simulink model "AdaptiveMPC"  (R2022b)
settings: Solver=VariableStepAuto  StartTime=0.0  StopTime=40  FixedStep=0.02  RelTol=1e-5
values from neighbouring files (symbols this model uses):
  Matlab_version = str2double(r_temp___(1))    [3T_articulation_soft_terrain.m]
  Plant_inputs_num = r_temp___(1)    [3T_articulation_soft_terrain.m]
  Plant_outputs_num = r_temp___(1)    [3T_articulation_soft_terrain.m]
  RecurDyn_controltimestep = 1.e-003    (= 0.001)    [3T_articulation_soft_terrain.m]
  RecurDyn_CoSim = 'D:\Program Files\FunctionBay, Inc\RecurDyn V9R1\Toolkits\Controls\Simulink30\'    [3T_articulation_soft_terrain.m]
  RecurDyn_model = '3T_articulation_soft_terrain'    [3T_articulation_soft_terrain.m]
  RecurDyn_model_n = r_temp___(2)    [3T_articulation_soft_terrain.m]
undefined symbols (not defined in the file or in its folder): magnitude, val
libraries: mpclib x2
settings Model: PacingRate=3  Creator=HU  LastModifiedBy=HU
settings DebuggingCC: UnconnectedInputMsg=warning  UnconnectedOutputMsg=warning  UnconnectedLineMsg=warning  SFMachineParentedDataDiag=warning
settings ModelReferenceCC: EnableRefExpFcnMdlSchedulingChecks=on
settings RTWCC: DLArmComputeVersion=19.05

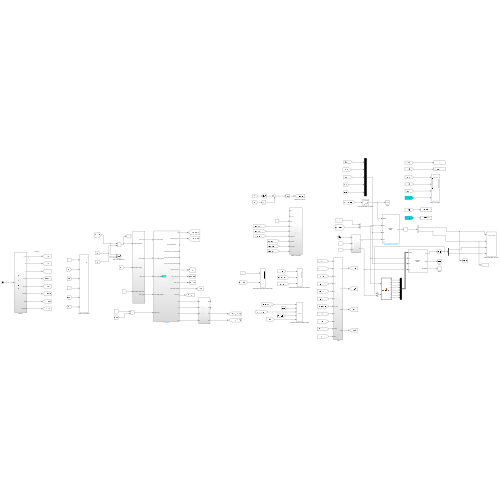
[thumbnail: Simulink's stored preview of the top-level diagram]
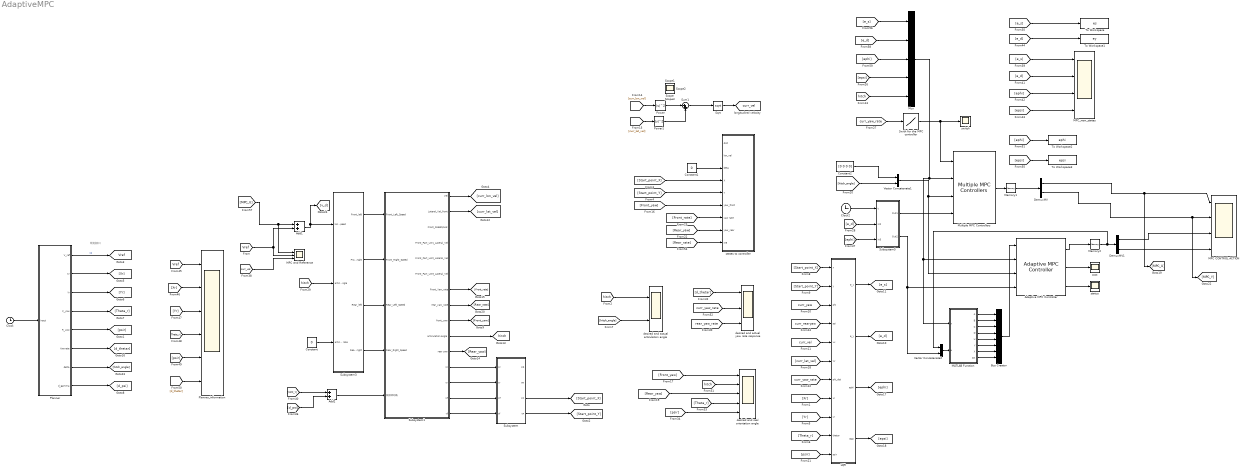
== system AdaptiveMPC ==
  note: 规划接口
  Adaptive MPC Controller : mpclib/Adaptive MPC Controller  SCDEnableBlockLinearizationSpecification=on  mpcobj=mpcobj_M_27  enable_value=0  updateMPCinCallerWorkspace=on  md_inport=on  mv_inport=off  uref_inport=off  return_cost=on  return_mvseq=off  return_qpstatus=on  return_xseq=off  return_state=off  return_ovseq=off  state_inport=off  isltv_plant=off  umin_inport=off  umax_inport=off  ymin_inport=off  ymax_inport=off  cc_inport=off  ywt_inport=off  uwt_inport=off  duwt_inport=off  rhoeps_inport=off  pm_inport=off  MaximumP=10  HorizonChoice=FixedHorizon  BlockDataType=double  SampleTimeInherited=off  switch_inport=off
  Add1 : Sum
  Add2 : Sum
  Bus Creator : BusCreator  Inputs=8
  Clock : Clock
  Clock2 : Clock
  Constant : Constant  Value=0
  Constant1 : Constant  Value=0
  Constant2 : Constant  Value=[0 0 0 0]
  DemuxMV : Demux  Outputs=2
  DemuxMV1 : Demux  Outputs=2
  LQR : Subsystem
  MATLAB Function : MATLAB Function  TreatAsAtomicUnit=on
  MPC CONTROL ACTION : Scope  NumInputPorts=4
  MPC and Reference : Scope  NumInputPorts=3
  MPC_new_states : Scope  NumInputPorts=4
  Memory1 : Memory
  Memory2 : Memory
  Multiple MPC Controllers : mpclib/Multiple MPC Controllers  mpcobjs={'mpcobj_L_21','mpcobj_M_21','mpcobj_H_21'}  x0s={'[]','[]','[]'}  Nmpc=1  theMPC=1  nmv=1  nmo=1  nmd=1  nts=1  md_inport_multiple=on  mv_inport_multiple=off  uref_inport_multiple=off  return_cost_multiple=off  return_mvseq_multiple=off  return_qpstatus_multiple=off  return_xseq_multiple=off  return_state_multiple=off  return_ovseq_multiple=off  state_inport_multiple=off  umin_inport_multiple=off  umax_inport_multiple=off  ymin_inport_multiple=off  ymax_inport_multiple=off  ywt_inport_multiple=off  uwt_inport_multiple=off  duwt_inport_multiple=off  rhoeps_inport_multiple=off  BlockDataType_multiple=double  SampleTimeInherited_multiple=off
  Mux : Mux  Inputs=5
  Planner : Subsystem
  Planner_information : Scope  NumInputPorts=6
  Power : Math  Operator=magnitude^2
  Power1 : Math  Operator=magnitude^2
  Sqrt : Sqrt
  Subsystem : Subsystem
  Subsystem1 : Subsystem
  Subsystem3 : Subsystem
  Subsystem5 : Subsystem
  Sum1 : Sum  Inputs=|++
  Swith for the MPC controller : Lookup_n-D  NumberOfTableDimensions=1  BreakpointsForDimension1="[-0.5  0  0.5]"  BreakpointsForDimension1FirstPoint=-0.1  BreakpointsForDimension1Spacing=0.1  Table="[1  2  3]"  InterpMethod=Nearest  InternalRulePriority=Speed  RndMeth=Simplest
  To Workspace : ToWorkspace  VariableName=es  SaveFormat=Timeseries  SampleTime=-1
  To Workspace1 : ToWorkspace  VariableName=ey  SaveFormat=Timeseries  SampleTime=-1
  To Workspace2 : ToWorkspace  VariableName=ephi  SaveFormat=Timeseries  SampleTime=-1
  To Workspace3 : ToWorkspace  VariableName=epsi  SaveFormat=Timeseries  SampleTime=-1
  Vector Concatenate1 : Concatenate
  Vector Concatenate2 : Concatenate  Mode=Multidimensional array  ConcatenateDimension=2
  cost : Scope
  desired and actual articulation angle : Scope  NumInputPorts=2
  desired and actual yaw rate response : Scope  NumInputPorts=3
  desired and real orientation angle : Scope  NumInputPorts=5
  states to controller : Subsystem
  status : Scope
  switch : Scope
  Scope{,1..3} (4 alike) : Scope
  tag scope: Vref=global, curr_vel=global, hitch=global
  wires:
  [Start_point_Y] -> states to controller/5(Y)
  LQR/2(e_y) -> [e_d]
  LQR/1(e_x) -> [e_s]
  Planner/1(V_ref) -> [Vref]  "vp"
  [Xr] -> LQR/8(xr)
  [Theta_r] -> LQR/10(thetar)
  Planner/4(F_yaw) -> [Theta_r]
  [curr_lat_vel] -> LQR/6(vy)
  Planner/3(Yr) -> [Yr]
  Sum1/1 -> Sqrt/1
  [curr_yaw_rate] -> LQR/7(phi_dot)
  [curr_vel] -> LQR/5(vx)
  [curr_yaw] -> LQR/3(phi)
  [Start_point_Y] -> LQR/2(y)
  [Start_point_X] -> LQR/1(x)
  [Yr] -> LQR/9(yr)
  Planner/2(Xr) -> [Xr]
  Power1/1 -> Sum1/2
  Constant1/1 -> states to controller/3(beta)
  Power/1 -> Sum1/1
  [Start_point_X] -> states to controller/4(X)
  Planner/6(Yawrate) -> [d_thetar]
  Planner/5(R_yaw) -> [psir]
  [psir] -> LQR/11(psir)
  [curr_rearyaw] -> LQR/4(psi)
  LQR/3(ephi) -> [ephi]
  LQR/4(epsi) -> [epsi]
  [d_thetar] -> desired and actual yaw rate response/1
  [Theta_r] -> desired and real orientation angle/4
  [psir] -> desired and real orientation angle/5
  [curr_yaw_rate] -> desired and actual yaw rate response/2
  [rear_yaw_rate] -> desired and actual yaw rate response/3
  [Front_yaw] -> desired and real orientation angle/1
  [Rear_yaw] -> desired and real orientation angle/3
  [e_s] -> MPC_new_states/1
  [e_d] -> MPC_new_states/2
  [ephi] -> MPC_new_states/3
  [epsi] -> MPC_new_states/4
  Subsystem1/2(Lateral_Vel_front) -> [curr_lat_vel]
  Subsystem3/1(Front_left) -> Subsystem1/1("Front_Left_Speed ")
  Subsystem3/2(Front_right) -> Subsystem1/2(Front_Right_Speed)
  Subsystem3/3(Rear_left) -> Subsystem1/3("Rear_Left_Speed  ")
  Subsystem3/4(Rear_right) -> Subsystem1/4("Rear_Right_Speed ")
  Subsystem1/12(Xr) -> Subsystem/1(Xr)
  Subsystem1/13(Yr) -> Subsystem/2(Yr)
  Subsystem1/14(Xf) -> Subsystem/3(Xf)
  Subsystem1/15(Yf) -> Subsystem/4(Yf)
  Subsystem1/1(Vel) -> [curr_lon_vel]
  [curr_lat_vel] -> Power1/1
  [curr_lon_vel] -> Power/1
  Subsystem1/9(front_yaw) -> [Front_yaw]
  [Front_yaw] -> states to controller/6(yaw_front)
  Subsystem1/11(rear yaw) -> [Rear_yaw]
  [Rear_yaw] -> states to controller/8(yaw_rear)
  Subsystem1/7(Front_Yaw_rate) -> [Front_rate]
  [Front_rate] -> states to controller/7(yaw rate)
  Subsystem1/8(rear_yaw_rate) -> [Rear_rate]
  Subsystem1/10(articulation angle) -> [hitch]
  [hitch] -> desired and real orientation angle/2
  [Vref] -> Planner_information/1
  [Yr] -> Planner_information/3
  [Theta_r] -> Planner_information/4
  [psir] -> Planner_information/5
  [d_thetar] -> Planner_information/6
  Planner/7(delta) -> [hitch_angle]
  [Xr] -> Planner_information/2
  Sqrt/1 -> [curr_vel]
  [hitch] -> Subsystem3/2(articulation angle)
  [Rear_rate] -> states to controller/9(In9)
  [ephi] -> Mux/3
  [hitch] -> Mux/5
  [e_d] -> Mux/2
  [e_s] -> Mux/1
  [MPC_U] -> Add1/1, MPC and Reference/1
  [Vref] -> Add1/2, MPC and Reference/2
  [epsi] -> Mux/4
  Mux/1 -> Multiple MPC Controllers/2, MATLAB Function/1(x), Adaptive MPC Controller/2
  Multiple MPC Controllers/1 -> Memory1/1
  Memory1/1 -> DemuxMV/1
  Swith for the MPC controller/1 -> Multiple MPC Controllers/1, switch/1
  Subsystem/4(YF) -> [Start_point_Y]
  Subsystem/3(XF) -> [Start_point_X]
  [hitch] -> desired and actual articulation angle/1
  [hitch_angle] -> desired and actual articulation angle/2
  Subsystem5/1(Out1) -> Multiple MPC Controllers/4
  [hitch_angle] -> Vector Concatenate1/2
  Constant2/1 -> Vector Concatenate1/1
  Clock2/1 -> Subsystem5/1(t)
  Vector Concatenate1/1 -> Multiple MPC Controllers/3, Adaptive MPC Controller/3
  MATLAB Function/1(A) -> Bus Creator/1
  MATLAB Function/2(B) -> Bus Creator/2
  MATLAB Function/3(C) -> Bus Creator/3
  MATLAB Function/4(D) -> Bus Creator/4
  MATLAB Function/5(U) -> Bus Creator/5
  MATLAB Function/6(Y) -> Bus Creator/6
  MATLAB Function/7(X) -> Bus Creator/7
  MATLAB Function/8(DX) -> Bus Creator/8
  Bus Creator/1 -> Adaptive MPC Controller/1
  Adaptive MPC Controller/1 -> Memory2/1
  DemuxMV1/1 -> MPC CONTROL ACTION/3
  DemuxMV1/2 -> MPC CONTROL ACTION/4
  Vector Concatenate2/1 -> MATLAB Function/2(u)
  Planner/8(d_gamma) -> [d_psi]
  [curr_yaw_rate] -> Swith for the MPC controller/1
  Memory2/1 -> Vector Concatenate2/1, DemuxMV1/1
  [e_d] -> Subsystem5/2(In2)
  [ephi] -> Subsystem5/3(In3)
  Adaptive MPC Controller/2 -> cost/1
  Adaptive MPC Controller/3 -> status/1
  [curr_vel] -> MPC and Reference/3
  Constant/1 -> Subsystem3/3(articulation angle rate)
  Add1/1 -> Subsystem3/1(longitudinal speed), [v_d]
  Subsystem5/2(Out2) -> Adaptive MPC Controller/4, Vector Concatenate2/2
  Clock/1 -> Planner/1(Input)
  [e_s] -> To Workspace/1
  [e_d] -> To Workspace1/1
  [ephi] -> To Workspace2/1
  [epsi] -> To Workspace3/1
  [MPC_Y] -> Add2/1
  Add2/1 -> Subsystem1/5("铰接转动角            ")
  [d_psi] -> Add2/2
  DemuxMV/1 -> [MPC_U], MPC CONTROL ACTION/1
  DemuxMV/2 -> [MPC_Y], MPC CONTROL ACTION/2

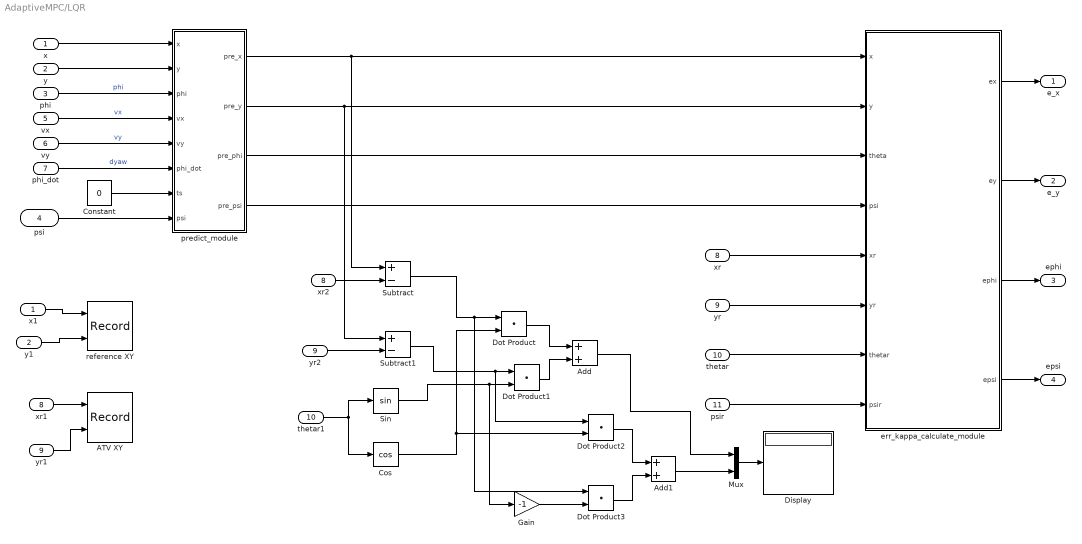
== system AdaptiveMPC/LQR ==
  x : Inport
  y : Inport  Port=2
  phi : Inport  Port=3
  psi : Inport  Port=4
  vx : Inport  Port=5
  vy : Inport  Port=6
  phi_dot : Inport  Port=7
  xr : Inport  Port=8
  yr : Inport  Port=9
  thetar : Inport  Port=10
  psir : Inport  Port=11
  ATV XY : Record  FileSettingsInternal="{\"entries\":[{\"content\":{\"excelSettings\":{\"content\":{},\"type\":\"Streamout.ExcelSettings\"}},\"type\":\"Streamout.FileSettingStorage\",\"uuid\":\"7d4ff071-c011-4d00-aaca-92aa85f924c6\"}],\"packageUris\":[\"http://schema.mathworks.com/mf0/streamout_blocks/R2020a\"],\"version\":\"1.0\"}"  Layout=[1 1]  SignalsInternal="{\"entries\":[{\"content\":{\"signals\":[{\"content\":{\"blockPath\":[\"AdaptiveMPC_only_MPC/LQR/ATV XY\"],\"channel\":[],\"dimensions\":[1],\"domain\":\"AdaptiveMPC_only_MPC/LQR/ATV XY\",\"lineColor\":\"#a2142f\",\"plots\":[1],\"port\":1,\"sid\":[\"\"],\"signalID\":165725,\"signalName\":\"xr1\"},\"type\":\"RecordBlkView.Signal\",\"uuid\":\"68c8aef4-2586-4868-bddc-4b1de75c0796\"},{\"content\":{\"blockPath\":[\"AdaptiveMPC_only_MPC/LQR/ATV XY\"],\"channel\":[],\"dimensions\":[1],\"domain\":\"AdaptiveMPC_only_MPC/LQR/ATV XY\",\"lineColor\":\"#139fff\",\"plots\":[1],\"port\":2,\"sid\":[\"\"],\"signalID\":165729,\"signalName\":\"yr1\"},\"type\":\"RecordBlkView.Signal\",\"uuid\":\"206c790a-a246-4103-b7c9-0af210733676\"}]},\"type\":\"RecordBlkView.InputSignals\",\"uuid\":\"6523171a-3a0a-4dbe-b18c-2b5d012fbce6\"}],\"packageUris\":[\"http://schema.mathworks.com/mf0/streamout_blocks/R2020a\"],\"version\":\"1.0\"}"  VisualizationBindings="{\"xyplotplugin\":{\"info\":[{\"series\":[{\"bindingParametersList\":[{\"parameter\":\"X-Axis\",\"signalID\":165725,\"signalName\":\"xr1\"},{\"parameter\":\"Y-Axis\",\"signalID\":165729,\"signalName\":\"yr1\"}],\"seriesID\":583}],\"subplotID\":1}]}}"  CompatibilityTag=XY  st=-1
  Add : Sum
  Add1 : Sum
  Constant : Constant  Value=0
  Cos : Trigonometry  Operator=cos
  Display : Display
  Dot Product{,1..3} (4 alike) : DotProduct  OutDataTypeStr=Inherit: Inherit via internal rule
  Gain : Gain  Gain=-1
  Mux : Mux  Inputs=2
  Sin : Trigonometry
  Subtract : Sum  Inputs=+-
  Subtract1 : Sum  Inputs=+-
  err_kappa_calculate_module : MATLAB Function  TreatAsAtomicUnit=on
  predict_module : MATLAB Function  TreatAsAtomicUnit=on
  reference XY : Record  FileSettingsInternal="{\"entries\":[{\"content\":{\"excelSettings\":{\"content\":{},\"type\":\"Streamout.ExcelSettings\"}},\"type\":\"Streamout.FileSettingStorage\",\"uuid\":\"01dd9b82-04e5-459d-9b91-d9a9579cc2c9\"}],\"packageUris\":[\"http://schema.mathworks.com/mf0/streamout_blocks/R2020a\"],\"version\":\"1.0\"}"  Layout=[1 1]  SignalsInternal="{\"entries\":[{\"content\":{\"signals\":[{\"content\":{\"blockPath\":[\"AdaptiveMPC_only_MPC/LQR/reference XY\"],\"channel\":[],\"dimensions\":[1],\"domain\":\"AdaptiveMPC_only_MPC/LQR/reference XY\",\"lineColor\":\"#a2142f\",\"plots\":[1],\"port\":1,\"sid\":[\"\"],\"signalID\":165733,\"signalName\":\"x1\"},\"type\":\"RecordBlkView.Signal\",\"uuid\":\"15320c6c-986b-4afd-bf62-20c31eac0383\"},{\"content\":{\"blockPath\":[\"AdaptiveMPC_only_MPC/LQR/reference XY\"],\"channel\":[],\"dimensions\":[1],\"domain\":\"AdaptiveMPC_only_MPC/LQR/reference XY\",\"lineColor\":\"#139fff\",\"plots\":[1],\"port\":2,\"sid\":[\"\"],\"signalID\":165737,\"signalName\":\"y1\"},\"type\":\"RecordBlkView.Signal\",\"uuid\":\"756ffe9f-769c-4c77-bafa-21ea174eeee0\"}]},\"type\":\"RecordBlkView.InputSignals\",\"uuid\":\"98c54ad5-dfe3-4874-ac3d-5744926d3a13\"}],\"packageUris\":[\"http://schema.mathworks.com/mf0/streamout_blocks/R2020a\"],\"version\":\"1.0\"}"  VisualizationBindings="{\"xyplotplugin\":{\"info\":[{\"series\":[{\"bindingParametersList\":[{\"parameter\":\"X-Axis\",\"signalID\":165733,\"signalName\":\"x1\"},{\"parameter\":\"Y-Axis\",\"signalID\":165737,\"signalName\":\"y1\"}],\"seriesID\":16425}],\"subplotID\":1}]}}"  CompatibilityTag=XY  st=-1
  thetar1 : InportShadow  Port=10
  x1 : InportShadow
  xr1 : InportShadow  Port=8
  xr2 : InportShadow  Port=8
  y1 : InportShadow  Port=2
  yr1 : InportShadow  Port=9
  yr2 : InportShadow  Port=9
  e_x : Outport  VectorParamsAs1DForOutWhenUnconnected=off
  e_y : Outport  Port=2  VectorParamsAs1DForOutWhenUnconnected=off
  ephi : Outport  Port=3  VectorParamsAs1DForOutWhenUnconnected=off
  epsi : Outport  Port=4  VectorParamsAs1DForOutWhenUnconnected=off
  wires:
  vy/1 -> predict_module/5(vy)  "vy"
  x/1 -> predict_module/1(x)
  predict_module/2(pre_y) -> Subtract1/1, err_kappa_calculate_module/2(y)
  phi_dot/1 -> predict_module/6(phi_dot)  "dyaw"
  vx/1 -> predict_module/4(vx)  "vx"
  y/1 -> predict_module/2(y)
  phi/1 -> predict_module/3(phi)  "phi"
  Constant/1 -> predict_module/7(ts)
  predict_module/1(pre_x) -> Subtract/1, err_kappa_calculate_module/1(x)
  predict_module/3(pre_phi) -> err_kappa_calculate_module/3(theta)
  xr/1 -> err_kappa_calculate_module/5(xr)
  yr/1 -> err_kappa_calculate_module/6(yr)
  thetar/1 -> err_kappa_calculate_module/7(thetar)
  psi/1 -> predict_module/8(psi)
  predict_module/4(pre_psi) -> err_kappa_calculate_module/4(psi)
  psir/1 -> err_kappa_calculate_module/8(psir)
  err_kappa_calculate_module/2(ey) -> e_y/1
  err_kappa_calculate_module/1(ex) -> e_x/1
  xr1/1 -> ATV XY/1
  yr1/1 -> ATV XY/2
  x1/1 -> reference XY/1
  y1/1 -> reference XY/2
  err_kappa_calculate_module/4(epsi) -> epsi/1
  err_kappa_calculate_module/3(ephi) -> ephi/1
  xr2/1 -> Subtract/2
  yr2/1 -> Subtract1/2
  thetar1/1 -> Cos/1, Sin/1
  Subtract/1 -> Dot Product/1, Dot Product3/1
  Cos/1 -> Dot Product2/2, Dot Product/2
  Subtract1/1 -> Dot Product2/1, Dot Product1/1
  Sin/1 -> Gain/1, Dot Product1/2
  Dot Product/1 -> Add/1
  Dot Product1/1 -> Add/2
  Gain/1 -> Dot Product3/2
  Dot Product2/1 -> Add1/1
  Dot Product3/1 -> Add1/2
  Add/1 -> Mux/1
  Add1/1 -> Mux/2
  Mux/1 -> Display/1

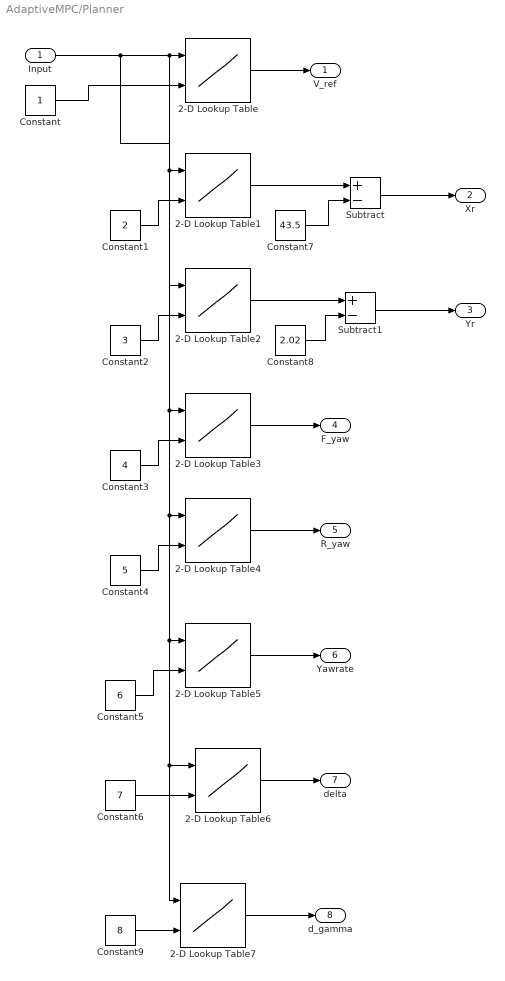
== system AdaptiveMPC/Planner ==
  Input : Inport
  2-D Lookup Table{,1..7} (8 alike) : Lookup_n-D  BreakpointsForDimension1=t  BreakpointsForDimension2=[1:8]  Table=val  InternalRulePriority=Speed  RndMeth=Simplest
      settings: InputPortMap=u0,u1
  Constant : Constant
  Constant1 : Constant  Value=2
  Constant2 : Constant  Value=3
  Constant3 : Constant  Value=4
  Constant4 : Constant  Value=5
  Constant5 : Constant  Value=6
  Constant6 : Constant  Value=7
  Constant7 : Constant  Value=43.5
  Constant8 : Constant  Value=2.02
  Constant9 : Constant  Value=8
  Subtract : Sum  Inputs=+-
  Subtract1 : Sum  Inputs=+-
  V_ref : Outport
  Xr : Outport  Port=2
  Yr : Outport  Port=3
  F_yaw : Outport  Port=4
  R_yaw : Outport  Port=5
  Yawrate : Outport  Port=6
  delta : Outport  Port=7
  d_gamma : Outport  Port=8
  wires:
  2-D Lookup Table6/1 -> delta/1
  Constant6/1 -> 2-D Lookup Table6/2
  Constant5/1 -> 2-D Lookup Table5/2
  2-D Lookup Table5/1 -> Yawrate/1
  Constant3/1 -> 2-D Lookup Table3/2
  Constant4/1 -> 2-D Lookup Table4/2
  2-D Lookup Table3/1 -> F_yaw/1
  Constant1/1 -> 2-D Lookup Table1/2
  2-D Lookup Table/1 -> V_ref/1
  Constant/1 -> 2-D Lookup Table/2
  Constant2/1 -> 2-D Lookup Table2/2
  Input/1 -> 2-D Lookup Table7/1, 2-D Lookup Table6/1, 2-D Lookup Table5/1, 2-D Lookup Table4/1, 2-D Lookup Table3/1, 2-D Lookup Table1/1, 2-D Lookup Table2/1, 2-D Lookup Table/1
  2-D Lookup Table4/1 -> R_yaw/1
  2-D Lookup Table1/1 -> Subtract/1
  Constant7/1 -> Subtract/2
  Subtract/1 -> Xr/1
  Subtract1/1 -> Yr/1
  Constant8/1 -> Subtract1/2
  2-D Lookup Table2/1 -> Subtract1/1
  Constant9/1 -> 2-D Lookup Table7/2
  2-D Lookup Table7/1 -> d_gamma/1

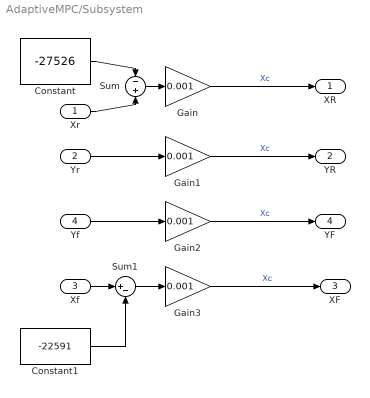
== system AdaptiveMPC/Subsystem ==
  Xr : Inport
  Yr : Inport  Port=2
  Xf : Inport  Port=3
  Yf : Inport  Port=4
  Constant : Constant  Value=-27526
  Constant1 : Constant  Value=-22591
  Gain{,1..3} (4 alike) : Gain  Gain=0.001
  Sum : Sum  Inputs=-+
  Sum1 : Sum  Inputs=|+-
  XR : Outport
  YR : Outport  Port=2
  XF : Outport  Port=3
  YF : Outport  Port=4
  wires:
  Gain/1 -> XR/1  "Xc"
  Xr/1 -> Sum/2
  Constant/1 -> Sum/1
  Sum/1 -> Gain/1
  Yr/1 -> Gain1/1
  Yf/1 -> Gain2/1
  Xf/1 -> Sum1/1
  Constant1/1 -> Sum1/2
  Sum1/1 -> Gain3/1
  Gain1/1 -> YR/1  "Xc"
  Gain3/1 -> XF/1  "Xc"
  Gain2/1 -> YF/1  "Xc"

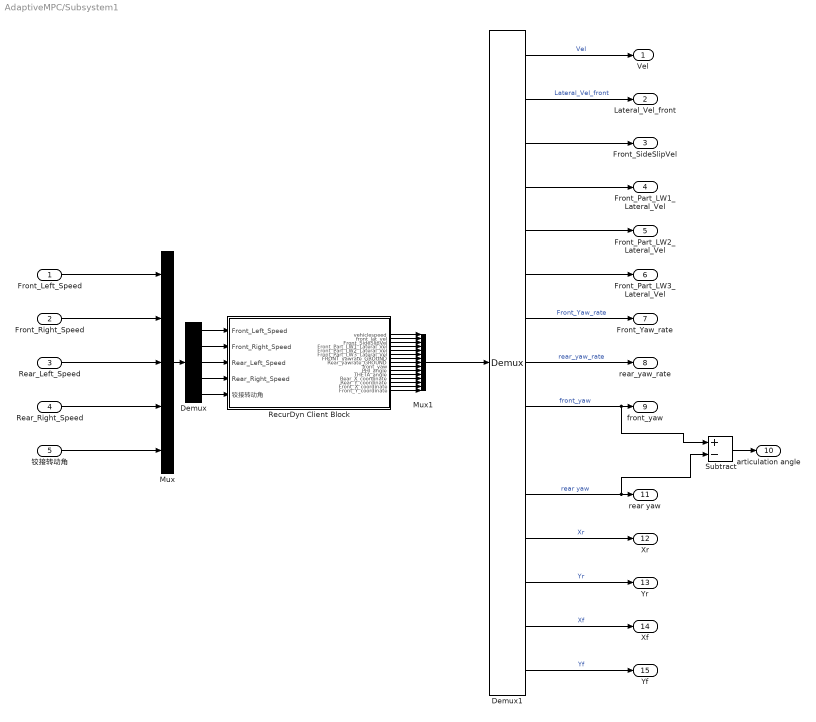
== system AdaptiveMPC/Subsystem1 ==
  "Front_Left_Speed " : Inport
  Front_Right_Speed : Inport  Port=2
  "Rear_Left_Speed  " : Inport  Port=3
  "Rear_Right_Speed " : Inport  Port=4
  "铰接转动角            " : Inport  Port=5
  Demux : Demux  Outputs=5
  Demux1 : Demux  Outputs=15
  Mux : Mux  Inputs=5
  Mux1 : Mux  Inputs=15
  RecurDyn Client Block : Subsystem
      mask Display: image(imread('RecurDyn_IF3x_Client.jpg'))
  Subtract : Sum  Inputs=+-
  Vel : Outport
  Lateral_Vel_front : Outport  Port=2
  "Front_SideSlipVel         " : Outport  Port=3
  Front_Part_LW1_Lateral_Vel : Outport  Port=4
  Front_Part_LW2_Lateral_Vel : Outport  Port=5
  Front_Part_LW3_Lateral_Vel : Outport  Port=6
  Front_Yaw_rate : Outport  Port=7
  rear_yaw_rate : Outport  Port=8
  front_yaw : Outport  Port=9
  articulation angle : Outport  Port=10
  rear yaw : Outport  Port=11
  Xr : Outport  Port=12
  Yr : Outport  Port=13
  Xf : Outport  Port=14
  Yf : Outport  Port=15
  wires:
  "Rear_Left_Speed  "/1 -> Mux/3
  Demux1/8 -> rear_yaw_rate/1  "rear_yaw_rate"
  Demux1/1 -> Vel/1  "Vel"
  Demux1/3 -> "Front_SideSlipVel         "/1
  Demux1/7 -> Front_Yaw_rate/1  "Front_Yaw_rate"
  Demux1/14 -> Xf/1  "Xf"
  Demux1/2 -> Lateral_Vel_front/1  "Lateral_Vel_front"
  Front_Right_Speed/1 -> Mux/2
  Demux1/13 -> Yr/1  "Yr"
  Demux1/12 -> Xr/1  "Xr"
  Demux1/15 -> Yf/1  "Yf"
  Demux1/4 -> Front_Part_LW1_Lateral_Vel/1
  "Front_Left_Speed "/1 -> Mux/1
  "Rear_Right_Speed "/1 -> Mux/4
  "铰接转动角            "/1 -> Mux/5
  Demux1/6 -> Front_Part_LW3_Lateral_Vel/1
  Demux1/5 -> Front_Part_LW2_Lateral_Vel/1
  Demux/1 -> RecurDyn Client Block/1("Front_Left_Speed ")
  Demux/2 -> RecurDyn Client Block/2(Front_Right_Speed)
  Demux/3 -> RecurDyn Client Block/3("Rear_Left_Speed  ")
  Demux/4 -> RecurDyn Client Block/4("Rear_Right_Speed ")
  Demux/5 -> RecurDyn Client Block/5("铰接转动角            ")
  Mux/1 -> Demux/1
  RecurDyn Client Block/1("vehiclespeed              ") -> Mux1/1
  RecurDyn Client Block/2("front_lat_vel             ") -> Mux1/2
  RecurDyn Client Block/3("Front_SideSlipVel         ") -> Mux1/3
  RecurDyn Client Block/4(Front_Part_LW1_Lateral_Vel) -> Mux1/4
  RecurDyn Client Block/5(Front_Part_LW2_Lateral_Vel) -> Mux1/5
  RecurDyn Client Block/6(Front_Part_LW3_Lateral_Vel) -> Mux1/6
  RecurDyn Client Block/7("FRONT_yawrate_GROUND      ") -> Mux1/7
  RecurDyn Client Block/8("Rear_yawrate_GROUND       ") -> Mux1/8
  RecurDyn Client Block/9("front_yaw                 ") -> Mux1/9
  RecurDyn Client Block/10("PHI_angle                 ") -> Mux1/10
  RecurDyn Client Block/11("THETA_angle               ") -> Mux1/11
  RecurDyn Client Block/12("Rear_X_coordinate         ") -> Mux1/12
  RecurDyn Client Block/13("Rear_Y_coordinate         ") -> Mux1/13
  RecurDyn Client Block/14("Front_X_coordinate        ") -> Mux1/14
  RecurDyn Client Block/15("Front_Y_coordinate        ") -> Mux1/15
  Mux1/1 -> Demux1/1
  Demux1/9 -> Subtract/1, front_yaw/1  "front_yaw"
  Demux1/11 -> Subtract/2, rear yaw/1  "rear yaw"
  Subtract/1 -> articulation angle/1

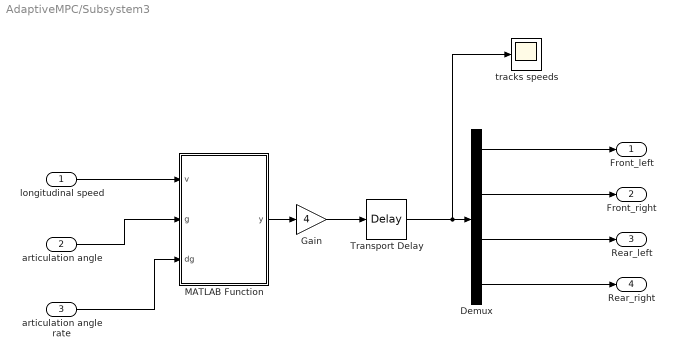
== system AdaptiveMPC/Subsystem3 ==
  longitudinal speed : Inport
  articulation angle : Inport  Port=2
  articulation angle rate : Inport  Port=3
  Demux : Demux
  Gain : Gain  Gain=4
  MATLAB Function : MATLAB Function  TreatAsAtomicUnit=on
  Transport Delay : TransportDelay  DelayTime=0.1
  tracks speeds : Scope
  Front_left : Outport
  Front_right : Outport  Port=2
  Rear_left : Outport  Port=3
  Rear_right : Outport  Port=4
  wires:
  articulation angle/1 -> MATLAB Function/2(g)
  MATLAB Function/1(y) -> Gain/1
  Gain/1 -> Transport Delay/1
  Demux/1 -> Front_left/1
  Demux/2 -> Front_right/1
  Demux/3 -> Rear_left/1
  Demux/4 -> Rear_right/1
  articulation angle rate/1 -> MATLAB Function/3(dg)
  Transport Delay/1 -> tracks speeds/1, Demux/1
  longitudinal speed/1 -> MATLAB Function/1(v)

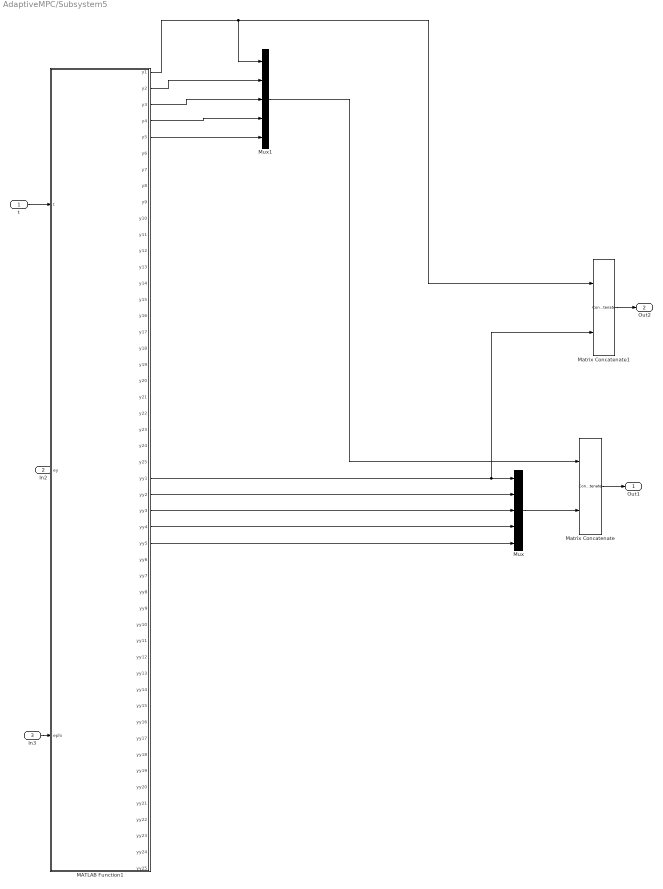
== system AdaptiveMPC/Subsystem5 ==
  t : Inport
  In2 : Inport  Port=2
  In3 : Inport  Port=3
  MATLAB Function1 : MATLAB Function  TreatAsAtomicUnit=on  SystemSampleTime=0.02
  Matrix Concatenate : Concatenate  Mode=Multidimensional array  ConcatenateDimension=2
  Matrix Concatenate1 : Concatenate  Mode=Multidimensional array  ConcatenateDimension=2
  Mux : Mux  Inputs=5
  Mux1 : Mux  Inputs=5
  Out1 : Outport
  Out2 : Outport  Port=2
  wires:
  MATLAB Function1/5(y5) -> Mux1/5
  Matrix Concatenate/1 -> Out1/1
  Mux/1 -> Matrix Concatenate/2
  MATLAB Function1/26(yy1) -> Matrix Concatenate1/2, Mux/1
  MATLAB Function1/29(yy4) -> Mux/4
  MATLAB Function1/3(y3) -> Mux1/3
  MATLAB Function1/4(y4) -> Mux1/4
  MATLAB Function1/1(y1) -> Matrix Concatenate1/1, Mux1/1
  MATLAB Function1/2(y2) -> Mux1/2
  MATLAB Function1/27(yy2) -> Mux/2
  MATLAB Function1/30(yy5) -> Mux/5
  MATLAB Function1/28(yy3) -> Mux/3
  Mux1/1 -> Matrix Concatenate/1
  t/1 -> MATLAB Function1/1(t)
  Matrix Concatenate1/1 -> Out2/1
  In2/1 -> MATLAB Function1/2(ey)
  In3/1 -> MATLAB Function1/3(ephi)

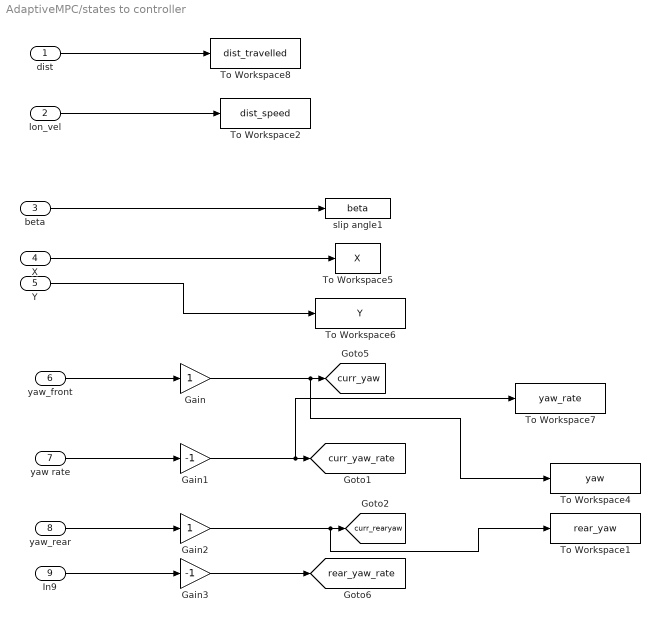
== system AdaptiveMPC/states to controller ==
  dist : Inport
  lon_vel : Inport  Port=2
  beta : Inport  Port=3
  X : Inport  Port=4
  Y : Inport  Port=5
  yaw_front : Inport  Port=6
  yaw rate : Inport  Port=7
  yaw_rear : Inport  Port=8
  In9 : Inport  Port=9
  Gain : Gain
  Gain1 : Gain  Gain=-1
  Gain2 : Gain
  Gain3 : Gain  Gain=-1
  To Workspace1 : ToWorkspace  VariableName=rear_yaw  SaveFormat=Timeseries  SampleTime=-1
  To Workspace2 : ToWorkspace  VariableName=dist_speed  SaveFormat=Timeseries  SampleTime=-1
  To Workspace4 : ToWorkspace  VariableName=yaw  SaveFormat=Timeseries  SampleTime=-1
  To Workspace5 : ToWorkspace  VariableName=X  SampleTime=-1
  To Workspace6 : ToWorkspace  VariableName=Y  SampleTime=-1
  To Workspace7 : ToWorkspace  VariableName=yaw_rate  SaveFormat=Timeseries  SampleTime=-1
  To Workspace8 : ToWorkspace  VariableName=dist_travelled  SaveFormat=Timeseries  SampleTime=-1
  slip angle1 : ToWorkspace  VariableName=beta  SaveFormat=Timeseries  SampleTime=-1
  tag scope: curr_rearyaw=global, curr_yaw=global, curr_yaw_rate=global, rear_yaw_rate=global
  wires:
  X/1 -> To Workspace5/1
  Y/1 -> To Workspace6/1
  beta/1 -> slip angle1/1
  yaw_front/1 -> Gain/1
  dist/1 -> To Workspace8/1
  lon_vel/1 -> To Workspace2/1
  yaw rate/1 -> Gain1/1
  Gain/1 -> To Workspace4/1, [curr_yaw]
  Gain1/1 -> To Workspace7/1, [curr_yaw_rate]
  Gain2/1 -> To Workspace1/1, [curr_rearyaw]
  yaw_rear/1 -> Gain2/1
  Gain3/1 -> [rear_yaw_rate]
  In9/1 -> Gain3/1

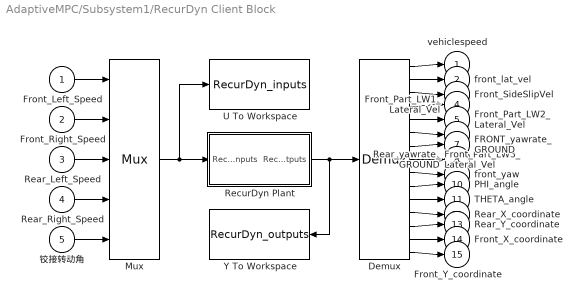
== system AdaptiveMPC/Subsystem1/RecurDyn Client Block ==
  "Front_Left_Speed " : Inport
  Front_Right_Speed : Inport  Port=2
  "Rear_Left_Speed  " : Inport  Port=3
  "Rear_Right_Speed " : Inport  Port=4
  "铰接转动角            " : Inport  Port=5
  Demux : Demux  Outputs=15
      settings: DisplayOption=none
  Mux : Mux  Inputs=5
  RecurDyn Plant : Subsystem  mask(Recurdyn/Plant){RecurDyn_model_name=RecurDyn_model, RecurDyn_controltimestep_=RecurDyn_controltimestep, RecurDyn_step_=10000, Waitingtime=1000, Matlab_version_=Matlab_version}
      mask prompts: RecurDyn_model_name "Model name"; RecurDyn_controltimestep_ "Sampling period"; RecurDyn_step_ "Step"; Waitingtime "Waiting time"; Matlab_version_ "Matlab version"
      mask help:
      | Simulate any Recurdyn Dynamics Model in Recurdyn/Solver
      | Plant inputs and Plant outputs are transfered every sampling time
      | Here, sampling time is determined by sampling period (Control time step)
      mask Display: disp( 'Dynamic Model' )
  U To Workspace : ToWorkspace  VariableName=RecurDyn_inputs
  Y To Workspace : ToWorkspace  VariableName=RecurDyn_outputs
  "vehiclespeed              " : Outport
  "front_lat_vel             " : Outport  Port=2
  "Front_SideSlipVel         " : Outport  Port=3
  Front_Part_LW1_Lateral_Vel : Outport  Port=4
  Front_Part_LW2_Lateral_Vel : Outport  Port=5
  Front_Part_LW3_Lateral_Vel : Outport  Port=6
  "FRONT_yawrate_GROUND      " : Outport  Port=7
  "Rear_yawrate_GROUND       " : Outport  Port=8
  "front_yaw                 " : Outport  Port=9
  "PHI_angle                 " : Outport  Port=10
  "THETA_angle               " : Outport  Port=11
  "Rear_X_coordinate         " : Outport  Port=12
  "Rear_Y_coordinate         " : Outport  Port=13
  "Front_X_coordinate        " : Outport  Port=14
  "Front_Y_coordinate        " : Outport  Port=15
  wires:
  "铰接转动角            "/1 -> Mux/5
  "Rear_Right_Speed "/1 -> Mux/4
  "Rear_Left_Speed  "/1 -> Mux/3
  Front_Right_Speed/1 -> Mux/2
  "Front_Left_Speed "/1 -> Mux/1
  Demux/15 -> "Front_Y_coordinate        "/1
  Demux/14 -> "Front_X_coordinate        "/1
  Demux/13 -> "Rear_Y_coordinate         "/1
  Demux/12 -> "Rear_X_coordinate         "/1
  Demux/11 -> "THETA_angle               "/1
  Demux/10 -> "PHI_angle                 "/1
  Demux/9 -> "front_yaw                 "/1
  Demux/8 -> "Rear_yawrate_GROUND       "/1
  Demux/7 -> "FRONT_yawrate_GROUND      "/1
  Demux/6 -> Front_Part_LW3_Lateral_Vel/1
  Demux/5 -> Front_Part_LW2_Lateral_Vel/1
  Demux/4 -> Front_Part_LW1_Lateral_Vel/1
  Demux/3 -> "Front_SideSlipVel         "/1
  Demux/2 -> "front_lat_vel             "/1
  Demux/1 -> "vehiclespeed              "/1
  Mux/1 -> U To Workspace/1, RecurDyn Plant/1(" RecurDyn_inputs")
  RecurDyn Plant/1(RecurDyn_outputs) -> Y To Workspace/1, Demux/1

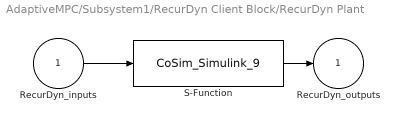
== system AdaptiveMPC/Subsystem1/RecurDyn Client Block/RecurDyn Plant ==
  " RecurDyn_inputs" : Inport
  S-Function : S-Function  FunctionName=CoSim_Simulink_9  Parameters=RecurDyn_controltimestep_,RecurDyn_model_name,RecurDyn_step_,Matlab_version_,RecurDyn_model_n,Plant_inputs_num,Plant_outputs_num,Waitingtime,RecurDyn_CoSim  SFunctionDeploymentMode=off  EnableBusSupport=off
  RecurDyn_outputs : Outport  InitialOutput=0
  wires:
  " RecurDyn_inputs"/1 -> S-Function/1
  S-Function/1 -> RecurDyn_outputs/1

== matlab function AdaptiveMPC/Subsystem3/MATLAB Function ==
  data: v input; y output; g input; dg input
function y = fcn(v, g, dg)
l=5;d=2.3;L1 = 2.6;L2 = 2.3; 
sg=sin(g); cg = L1+cos(g)*L2;c_g = 2*(L2+L1*cos(g));
t12 = v*sg/(2*cg);
t13 = v*dg*d*L1/(2*cg);
t21 = v*cos(g);
t22 = v*sg^2*L2/(c_g);
t23 = v*d*sg/c_g;
t24 = v*dg*L2*(2*L2*sg-d*cos(g))/c_g;
t25 = v*dg*L2*(2*L2*sg+d*cos(g))/c_g;
% y=[v+t12-t13;
%     v-t12+t13;
%     t21+t22+t23+t24;
%     t21+t22-t23+t25];
y  = [v;
      v;
      v*cos(g);
      v*cos(g)];

== matlab function AdaptiveMPC/MATLAB Function ==
  data: x input; u input; A output; B output; C output; D output; U output size=[4 1]; Y output size=[5 1]; X output size=[5 1]; DX output size=[5 1]
function [A,B,C,D,U,Y,X,DX] = adaptive_ATV(x,u)
[A,B,C,D,U,Y,X,DX] = ArticulatedVehicleModelDT32(x,u);

== matlab function AdaptiveMPC/LQR/err_kappa_calculate_module ==
  data: x input; y input; theta input; psi input; xr input; yr input; thetar input; ex output; ey output; ephi output; epsi output; psir input
function [ex,ey,ephi,epsi] = fcn(x,y,theta,psi,xr,yr,thetar,psir)
    
    tor=[cos(thetar);sin(thetar)];
    nor=[-sin(thetar);cos(thetar)];
    d_err=[x-xr;y-yr];
    ex=tor'*d_err;
    ey=nor'*d_err;

    %%%%%%%%%
    ephi = theta-thetar;
    epsi = psi-psir;
    %%%%%%%%%
    
    
    
    
    
    
    
    
    
    
    


end

== matlab function AdaptiveMPC/LQR/predict_module ==
  data: x input; pre_x output; y input; phi input; vx input; vy input; phi_dot input; ts input; pre_y output; pre_phi output; pre_psi output; psi input
function [pre_x,pre_y,pre_phi,pre_psi] = fcn(x,y,phi,vx,vy,phi_dot,ts, psi)
    pre_x=x+vx*ts*cos(phi)-vy*ts*sin(phi);
    pre_y=y+vy*ts*cos(phi)+vx*ts*sin(phi);
    pre_phi=phi+phi_dot*ts;
    pre_psi = psi + phi_dot*ts;
end

== matlab function AdaptiveMPC/Subsystem5/MATLAB Function1 ==
  data: t input double size=1; y1 output; y2 output; y3 output; y4 output; y5 output; y6 output; y7 output; y8 output; y9 output; y10 output; y11 output; y12 output; y13 output; y14 output; y15 output; y16 output; y17 output; y18 output; y19 output; y20 output; y21 output; y22 output; y23 output; y24 output; y25 output; yy1 output; yy2 output; yy3 output; yy4 output; yy5 output; yy6 output; yy7 output; yy8 output; yy9 output; yy10 output; yy11 output; yy12 output; yy13 output; yy14 output; yy15 output; yy16 output; yy17 output; yy18 output; yy19 output; yy20 output; yy21 output; yy22 output; yy23 output; yy24 output; yy25 output; ey input; ephi input
function [y1, y2, y3, y4, y5, y6, y7, y8, y9, y10, y11, y12, y13, y14, y15, y16, y17,y18, y19, y20, y21, y22, y23, y24, y25, yy1, yy2, yy3, yy4 ,yy5 ,yy6 ,yy7 ,yy8 ,yy9, yy10, yy11, yy12, yy13 ,yy14 ,yy15,yy16 ,yy17 ,yy18 ,yy19, yy20, yy21, yy22, yy23 ,yy24 ,yy25] = vel_read(t,ey,ephi)
 t_data = load('F:\Recurdyn_simulation\mpc_cosimulation\mpc_result\311\t_total.mat');
 in   = load('F:\Recurdyn_simulation\mpc_cosimulation\mpc_result\311\planned_path.mat');
 time = t_data.t;
 val  = in.val;
 x = val(:,1);
 y = interp1(time,x,t:0.02:(t+0.02*24));
 y1 = y(1);
 y2 = y(2);
 y3 = y(3);
 y4 = y(4);
 y5 = y(5);
 y6 = y(6);
 y7 = y(7);
 y8 = y(8);
 y9 = y(9);
 y10 =y(10);
 y11 =y(11);
 y12 = y(12);
 y13 = y(13);
 y14 =y(14);
 y15 = y(15);
 y16 =y(16);
 
 y17 = y(17);
 y18 = y(18);
 y19 = y(19);
 y20 =y(20);
 y21 =y(21);
 y22 = y(22);
 y23 = y(23);
 y24 =y(24);
 y25 = y(25);

 xx = val(:,6);
 yy = interp1(time,xx,t:0.02:(t+0.02*24));
 yy1 = yy(1);
 yy2 = yy(2);
 yy3 = yy(3);
 yy4 = yy(4);
 yy5 = yy(5);
 yy6 = yy(6);
 yy7 = yy(7);
 yy8 = yy(8);
 yy9 = yy(9);
 yy10 =yy(10);
 yy11 =yy(11);
 yy12 = yy(12);
 yy13 = yy(13);
 yy14 =yy(14);
 yy15 = yy(15);
 yy16 =yy(16);
 
 yy17 = yy(17);
 yy18 = yy(18);
 yy19 = yy(19);
 yy20 =yy(20);
 yy21 =yy(21);
 yy22 = yy(22);
 yy23 = yy(23);
 yy24 =yy(24);
 yy25 = yy(25);
end
